simulink model "Diagrama_desaladoras_PSA"  (R2019b)
settings: Solver=VariableStepAuto  StartTime=0.0  StopTime=10.0  RelTol=1e-3
libraries: Libreria x12
settings Model: Creator=PC-01  LastModifiedBy=PC-01

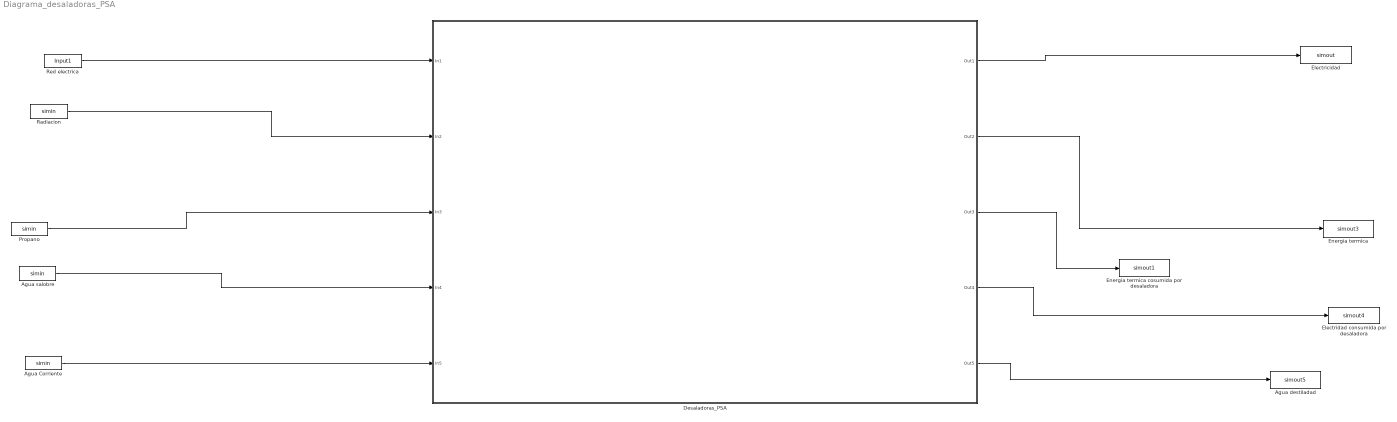
== system Diagrama_desaladoras_PSA ==
  Agua Corriente : FromWorkspace  VariableName=simin  SampleTime=0
  Agua destiladad : ToWorkspace  VariableName=simout5  SaveFormat=Timeseries  SampleTime=-1
  Agua salobre : FromWorkspace  VariableName=simin  SampleTime=0
  Desaladoras_PSA : Subsystem
  Electricidad : ToWorkspace  VariableName=simout  SaveFormat=Timeseries  SampleTime=-1
  Electridad consumida por desaladora : ToWorkspace  VariableName=simout4  SaveFormat=Timeseries  SampleTime=-1
  Energia termica : ToWorkspace  VariableName=simout3  SaveFormat=Timeseries  SampleTime=-1
  Energia termica cosumida por desaladora : ToWorkspace  VariableName=simout1  SaveFormat=Timeseries  SampleTime=-1
  Propano : FromWorkspace  VariableName=simin  SampleTime=0
  Radiacion : FromWorkspace  VariableName=simin  SampleTime=0
  Red electrica : FromWorkspace  VariableName=Input1  SampleTime=0
  wires:
  Red electrica/1 -> Desaladoras_PSA/1(In1)
  Radiacion/1 -> Desaladoras_PSA/2(In2)
  Propano/1 -> Desaladoras_PSA/3(In3)
  Agua salobre/1 -> Desaladoras_PSA/4(In4)
  Agua Corriente/1 -> Desaladoras_PSA/5(In5)
  Desaladoras_PSA/1(Out1) -> Electricidad/1
  Desaladoras_PSA/2(Out2) -> Energia termica/1
  Desaladoras_PSA/3(Out3) -> Energia termica cosumida por desaladora/1
  Desaladoras_PSA/4(Out4) -> Electridad consumida por desaladora/1
  Desaladoras_PSA/5(Out5) -> Agua destiladad/1

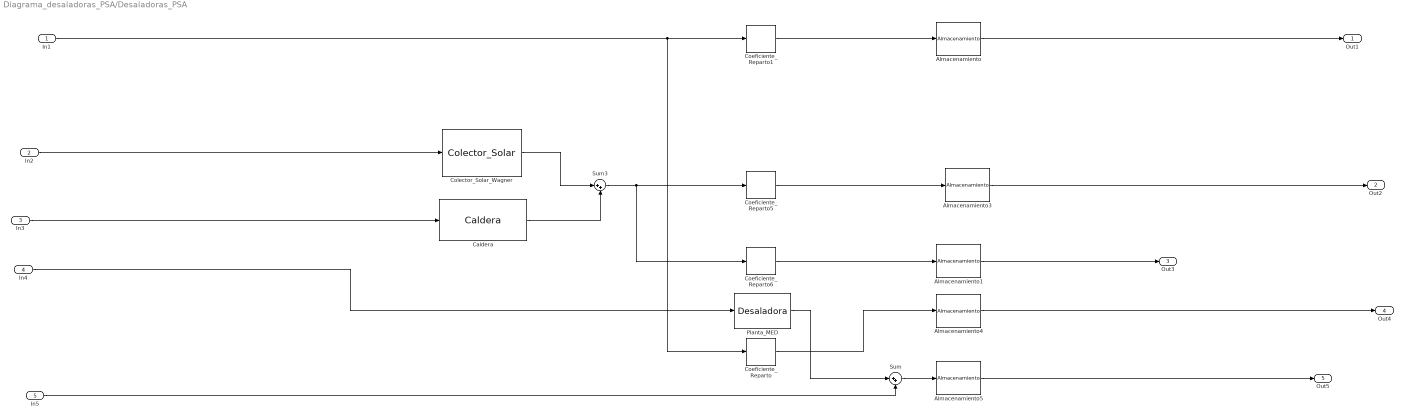
== system Diagrama_desaladoras_PSA/Desaladoras_PSA ==
  In1 : Inport
  In2 : Inport  Port=2
  In3 : Inport  Port=3
  In4 : Inport  Port=4
  In5 : Inport  Port=5
  Almacenamiento : Libreria/Almacenamiento  Up2=3  Low2=0  r_c=0.7  Up=3  Low=0  r_d=0.8  Up1=20  Low1=0  almacenamiento_inicial=0  cpa=0.02  almacenamiento_on=on
  Almacenamiento1 : Libreria/Almacenamiento  Up2=250.8  Low2=0  r_c=0.9  Up=250.8  Low=0  r_d=0.9  Up1=335.4  Low1=0  almacenamiento_inicial=0  cpa=0.06  almacenamiento_on=on
  Almacenamiento3 : Libreria/Almacenamiento  Up2=250.8  Low2=0  r_c=0.9  Up=250.8  Low=0  r_d=0.9  Up1=335.4  Low1=0  almacenamiento_inicial=0  cpa=0.06  almacenamiento_on=on
  Almacenamiento4 : Libreria/Almacenamiento  Up2=0  Low2=0  r_c=0  Up=0  Low=0  r_d=0  Up1=0  Low1=0  almacenamiento_inicial=0  cpa=1  almacenamiento_on=on
  Almacenamiento5 : Libreria/Almacenamiento  Up2=1000  Low2=0  r_c=1  Up=1000  Low=0  r_d=1  Up1=1000  Low1=0  almacenamiento_inicial=0  cpa=1  almacenamiento_on=on
  Caldera : Libreria/Caldera  efficiency=11.54  dispatch_factor=1  T_muestreo=T_muestreo  Min_in=0  Max_in=20  Max_out=230.8
  Coeficiente_Reparto{,1,5..6} (4 alike) : Libreria/Coeficiente_Reparto  dispatch_factor=1  Tm=T_muestreo  Max_out=inf  Max_in=inf  efficiency=1
  Colector_Solar_Wagner : Libreria/Colector_Solar  efficiency=0.59  dispatch_factor=1  T_muestreo=T_muestreo  Max_in=547.5  Max_out=323
  Planta_MED : Libreria/Desaladora  efficiency=0.32  dispatch_factor=beta1  T_muestreo=T_muestreo  Max_in=150  Max_out=150  n_salida=[3 4]
  Sum : Sum  Inputs=|++
  Sum3 : Sum  Inputs=|++
  Out1 : Outport
  Out2 : Outport  Port=2
  Out3 : Outport  Port=3
  Out4 : Outport  Port=4
  Out5 : Outport  Port=5
  wires:
  Coeficiente_Reparto5/1 -> Almacenamiento3/1
  Colector_Solar_Wagner/1 -> Sum3/1
  Almacenamiento3/1 -> Out2/1
  Almacenamiento5/1 -> Out5/1
  Coeficiente_Reparto6/1 -> Almacenamiento1/1
  Sum3/1 -> Coeficiente_Reparto6/1, Coeficiente_Reparto5/1
  Caldera/1 -> Sum3/2
  Coeficiente_Reparto1/1 -> Almacenamiento/1
  In1/1 -> Coeficiente_Reparto/1, Coeficiente_Reparto1/1
  Coeficiente_Reparto/1 -> Almacenamiento4/1
  In4/1 -> Planta_MED/1
  Sum/1 -> Almacenamiento5/1
  Planta_MED/1 -> Sum/1
  In2/1 -> Colector_Solar_Wagner/1
  Almacenamiento4/1 -> Out4/1
  Almacenamiento1/1 -> Out3/1
  In5/1 -> Sum/2
  Almacenamiento/1 -> Out1/1
  In3/1 -> Caldera/1
